simulink model "Test_PQ_Control_LCL_4Legs"  (R2023b)
settings: Solver=VariableStepAuto  StartTime=0.0  StopTime=5  RelTol=1e-3
InitFcn:
  | %Initialization_for_ESS_3P_2L_220kW;
values from neighbouring files (symbols this model uses):
  C_grid = 54e-6    (= 5.4e-05)    [Initialization_for_ESS_3P_2L_220kW.m]    (also in Initialization_for_Testbench.m = 4.5e-05)
  Cdc = 180e-6    (= 0.00018)    [CurrentLoop.m]    (also in Initialization_for_ESS_3P_2L_220kW.m; Initialization_for_Testbench.m)
  Fnom_Grid = 50    [CurrentLoop.m]    (also in Initialization_for_ESS_3P_2L_220kW.m; Initialization_for_Testbench.m)
  L_grid = 200e-6    (= 0.0002)    [Initialization_for_ESS_3P_2L_220kW.m]    (also in Initialization_for_Testbench.m)
  Ts_Control = 62.5e-6    (= 6.25e-05)    [CurrentLoop.m]    (also in Initialization_for_ESS_3P_2L_220kW.m; Initialization_for_Testbench.m = 0.0001)
  Ts_Power = 10e-7    (= 1e-06)    [Initialization_for_ESS_3P_2L_220kW.m]    (also in Initialization_for_Testbench.m)
  Udc_ref = 1500    [CurrentLoop.m]    (also in Initialization_for_ESS_3P_2L_220kW.m; Initialization_for_Testbench.m)
  Unom_Grid = 690    [CurrentLoop.m]    (also in Initialization_for_ESS_3P_2L_220kW.m; Initialization_for_Testbench.m)
undefined symbols (not defined in the file or in its folder): L_neutral
libraries: spsSeriesRLCBranchLib x4, spsThreePhaseVIMeasurementLib x4, simulink x3, spsTriangleGeneratorLib x3, spsThreePhaseSeriesRLCBranchLib x3, spsMultimeterLib x2, spsThreePhaseSeriesRLCLoadLib x2, spsThreePhaseBreakerLib x2, spsUniversalBridgeLib x2, eeStairGenerator x1, spsDCVoltageSourceLib x1, spsRMSLib x1
settings Model: Creator=ZZY  LastModifiedBy=ZZY
settings DataIOCC: ReturnWorkspaceOutputs=off
settings OptimizationCC: UseDivisionForNetSlopeComputation=on

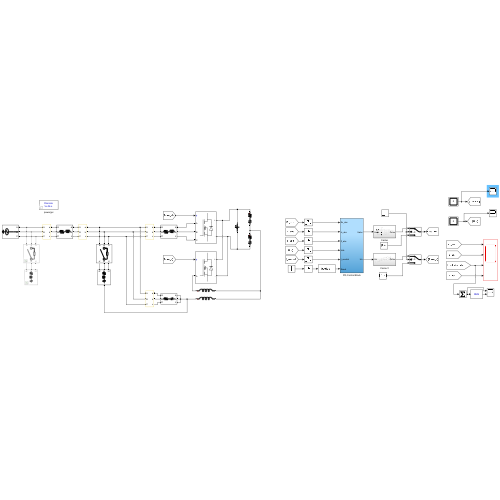
[thumbnail: Simulink's stored preview of the top-level diagram]
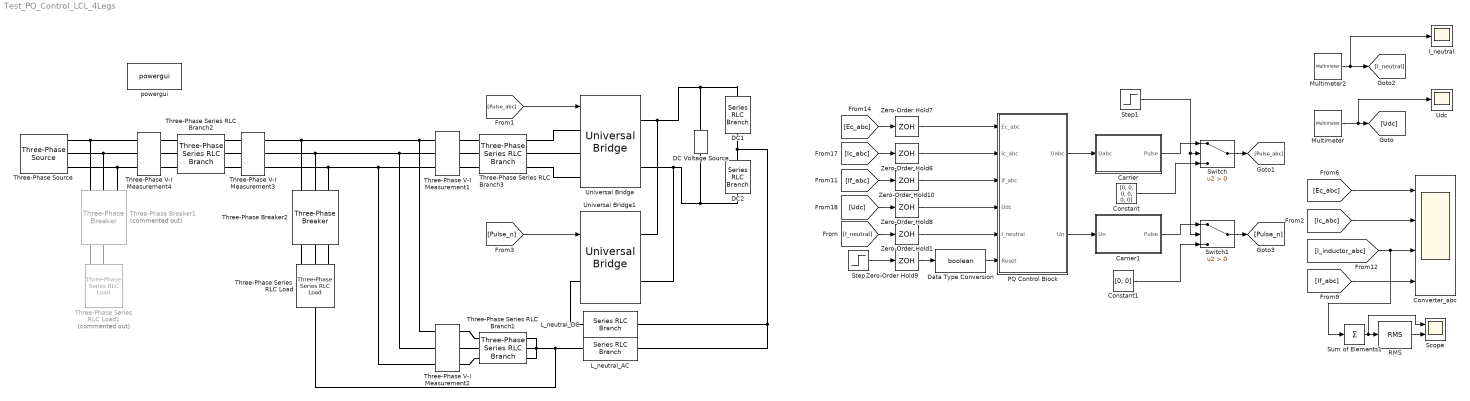
== system Test_PQ_Control_LCL_4Legs ==
  " PQ Control Block" : Subsystem
  Carrier : Subsystem
  Carrier1 : Subsystem
  Constant : Constant  Value=[0, 0, 0, 0, 0, 0]
  Constant1 : Constant  Value=[0, 0]
  Converter_abc : Scope  NumInputPorts=4
  DC Voltage Source : spsDCVoltageSourceLib/DC Voltage Source  Amplitude=Udc_ref  Measurements=None
  DC1 : spsSeriesRLCBranchLib/Series RLC Branch  LConnTagsString=__new0  RConnTagsString=__new0  BranchType=RC  Resistance=1e-4  Inductance=1e-3  SetiL0=off  InitialCurrent=0  Capacitance=Cdc*1.1  Setx0=on  InitialVoltage=Udc_ref/3  Measurements=Branch voltage
  DC2 : spsSeriesRLCBranchLib/Series RLC Branch  LConnTagsString=__new0  RConnTagsString=__new0  BranchType=RC  Resistance=1e-4  Inductance=1e-3  SetiL0=off  InitialCurrent=0  Capacitance=Cdc*0.9  Setx0=on  InitialVoltage=Udc_ref/2  Measurements=Branch voltage
  Data Type Conversion : DataTypeConversion  OutDataTypeStr=boolean  SaturateOnIntegerOverflow=off  RndMeth=Floor
  I_neutral : Scope
  L_neutral_AC : spsSeriesRLCBranchLib/Series RLC Branch  LConnTagsString=__new0  RConnTagsString=__new0  BranchType=L  Resistance=1e-6  Inductance=100e-6  SetiL0=off  InitialCurrent=0  Capacitance=Cdc  Setx0=on  InitialVoltage=750  Measurements=Branch current
  L_neutral_DC : spsSeriesRLCBranchLib/Series RLC Branch  LConnTagsString=__new0  RConnTagsString=__new0  BranchType=L  Resistance=L_neutral  Inductance=L_neutral  SetiL0=off  InitialCurrent=0  Capacitance=Cdc  Setx0=on  InitialVoltage=750  Measurements=Branch current
  Multimeter : spsMultimeterLib/Multimeter  L=4  sel=[1 2]  yselected={}  Gain=[1 1]  OutputType=Complex  PlotAtSimulationStop=off  PhasorSimulation=off
  Multimeter2 : spsMultimeterLib/Multimeter  L=4  sel=[3 4]  yselected={}  Gain=[1 1]  OutputType=Complex  PlotAtSimulationStop=off  PhasorSimulation=off
  RMS : spsRMSLib/RMS  TrueRMS=on  Freq=100  RMSInit=0  Ts=0
  Scope : Scope  NumInputPorts=2
  Step : Step  Time=0.5  OutDataTypeStr=Inherit: Inherit via back propagation  SampleTime=Ts_Control
  Step1 : Step  Time=0.01  OutDataTypeStr=Inherit: Inherit via back propagation  SampleTime=Ts_Control
  Sum of Elements1 : Sum  Inputs=+
  Switch : Switch  Criteria=u2 > Threshold  SaturateOnIntegerOverflow=off  InputSameDT=off
  Switch1 : Switch  Criteria=u2 > Threshold  SaturateOnIntegerOverflow=off  InputSameDT=off
  Three-Phase Series RLC Branch1 : spsThreePhaseSeriesRLCBranchLib/Three-Phase Series RLC Branch  LConnTagsString=A|B|C  RConnTagsString=A|B|C  BranchType=RC  Resistance=10e-3  Inductance=1e-3  Capacitance=C_grid  Measurements=None
  Three-Phase Series RLC Branch2 : spsThreePhaseSeriesRLCBranchLib/Three-Phase Series RLC Branch  LConnTagsString=A|B|C  RConnTagsString=A|B|C  BranchType=RL  Resistance=1e-6  Inductance=L_grid*1  Capacitance=1e-6  Measurements=None
  Three-Phase Series RLC Branch3 : spsThreePhaseSeriesRLCBranchLib/Three-Phase Series RLC Branch  LConnTagsString=A|B|C  RConnTagsString=A|B|C  BranchType=RL  Resistance=1e-6  Inductance=L_grid  Capacitance=1e-6  Measurements=None
  Three-Phase Series RLC Load : spsThreePhaseSeriesRLCLoadLib/Three-Phase Series RLC Load  LConnTagsString=A|B|C  RConnTagsString=N  Configuration=Y (neutral)  NominalVoltage=690  Vabc=[400 400 400]  Vabcp=[1e3 1e3 1e3]  NominalFrequency=50  UnbalancedPower=on  ActivePower=100e3  InductivePower=50e3  CapacitivePower=0  Pabc=[10e3 9e3 11e3]  QLabc=[10 90 110]  QCabc=[100 90 110]  Pabcp=[10e3 9e3 11e3]  QLabcp=[100 90 110]  QCabcp=[100 90 110]  Measurements=None  LoadType=constant Z
  Three-Phase Series RLC Load1 : spsThreePhaseSeriesRLCLoadLib/Three-Phase Series RLC Load  Commented=on  LConnTagsString=A|B|C  Configuration=Delta  NominalVoltage=690  Vabc=[400 400 400]  Vabcp=[1e3 1e3 1e3]  NominalFrequency=50  UnbalancedPower=on  ActivePower=100e3  InductivePower=50e3  CapacitivePower=0  Pabc=[10e3 9e3 11e3]  QLabc=[10 90 110]  QCabc=[100 90 110]  Pabcp=[10e3 9e3 11e3]  QLabcp=[100 90 110]  QCabcp=[100 90 110]  Measurements=None  LoadType=constant Z
  Three-Phase V-I Measurement1 : spsThreePhaseVIMeasurementLib/Three-Phase V-I Measurement  VoltageMeasurement=no  SetLabelV=on  LabelV=Ec_abc  Vpu=off  VpuLL=off  CurrentMeasurement=yes  SetLabelI=on  LabelI=I_inductor_abc  Ipu=off  Pbase=100e6  Vbase=500e3  OutputType=Complex  PhasorSimulation=off  PSBequivalent=0
  Three-Phase V-I Measurement2 : spsThreePhaseVIMeasurementLib/Three-Phase V-I Measurement  VoltageMeasurement=no  SetLabelV=off  LabelV=Ec_abc  Vpu=off  VpuLL=off  CurrentMeasurement=yes  SetLabelI=on  LabelI=If_abc  Ipu=off  Pbase=100e6  Vbase=500e3  OutputType=Complex  PhasorSimulation=off  PSBequivalent=0
  Three-Phase V-I Measurement3 : spsThreePhaseVIMeasurementLib/Three-Phase V-I Measurement  VoltageMeasurement=phase-to-phase  SetLabelV=on  LabelV=Ec_abc  Vpu=off  VpuLL=off  CurrentMeasurement=yes  SetLabelI=on  LabelI=Ic_abc  Ipu=off  Pbase=100e6  Vbase=500e3  OutputType=Complex  PhasorSimulation=off  PSBequivalent=0
  Three-Phase V-I Measurement4 : spsThreePhaseVIMeasurementLib/Three-Phase V-I Measurement  VoltageMeasurement=phase-to-phase  SetLabelV=on  LabelV=Eg_abc  Vpu=off  VpuLL=off  CurrentMeasurement=no  SetLabelI=on  LabelI=Ic_abc  Ipu=off  Pbase=100e6  Vbase=500e3  OutputType=Complex  PhasorSimulation=off  PSBequivalent=0
  Three-Phase Breaker1 : spsThreePhaseBreakerLib/Three-Phase Breaker  Commented=on  InitialState=open  SwitchA=on  SwitchB=on  SwitchC=on  SwitchTimes="[0.9  2.5]"  External=off  BreakerResistance=0.01  SnubberResistance=1e6  SnubberCapacitance=inf  Measurements=None
  Three-Phase Breaker2 : spsThreePhaseBreakerLib/Three-Phase Breaker  InitialState=open  SwitchA=on  SwitchB=on  SwitchC=on  SwitchTimes="[0.9  2.3]"  External=off  BreakerResistance=0.01  SnubberResistance=1e6  SnubberCapacitance=inf  Measurements=None
  Three-Phase Source : spsThreePhaseSourceLib/Three-Phase Source  InternalConnection=Yg  VoltagePhases=off  Voltage=Unom_Grid  PhaseAngle=0  Voltage_phases=[25e3 25e3 25e3]/sqrt(3)  PhaseAngles_phases=[0 -120 +120]  Frequency=Fnom_Grid  NonIdealSource=off  SpecifyImpedance=off  Resistance=1e-3  Inductance=400e-6  ShortCircuitLevel=100e6  BaseVoltage=Unom_Grid  XRratio=7  BusType=swing  Pref=10e3  Qref=0  Prefabc=[10e3, 10e3, 10e3]  Qrefabc=[0, 0, 0]  Qmin=-inf  Qmax=inf
  Udc : Scope
  Universal Bridge : spsUniversalBridgeLib/Universal Bridge  Arms=3  SnubberResistance=1e5  SnubberCapacitance=inf  Device=MOSFET / Diodes  Ron=1e-3  Lon=0  ForwardVoltages="[  0  0  ]"  ForwardVoltage=0  GTOparameters=[ 10e-6 , 20e-6 ]  IGBTparameters=[ 1e-6 , 2e-6 ]  Measurements=None  Measurements_2=None  converterType=Rectifier
  Universal Bridge1 : spsUniversalBridgeLib/Universal Bridge  Arms=1  SnubberResistance=1e5  SnubberCapacitance=inf  Device=MOSFET / Diodes  Ron=1e-3  Lon=0  ForwardVoltages="[  0  0  ]"  ForwardVoltage=0  GTOparameters=[ 10e-6 , 20e-6 ]  IGBTparameters=[ 1e-6 , 2e-6 ]  Measurements=None  Measurements_2=None  converterType=Rectifier
  Zero-Order Hold{1,6..10} (6 alike) : ZeroOrderHold  SampleTime=Ts_Control
  powergui : spspowerguiLib/powergui  Priority=1  SimulationMode=Discrete  SampleTime=Ts_Power  frequency=60  Iterations=50  frequencyindice=50  Pbase=100e6  ErrMax=1e-4  UnitsV=kV  UnitsW=MW  buscounter=0  FunctionMessages=off  echomessages=off  EnableUseOfTLC=off  CurrentSourceSwitches=off  DisableSnubberDevices=off  DisableRonSwitches=off  DisableVfSwitches=off  DisplayEquations=off  AutomaticDiscreteSolvers=off  SolverType=Tustin/Backward Euler (TBE)  Interpol=off  ExternalGateDelay=off  methode=off  Ts=100  x0status=blocks  SPID=on  SwTol=0  HookPort=off  NonlinearTolerance=1e-4  nMaxIteration=100  ContinueOnMaxIteration=off  RestoreLinks=warning  ResistiveCurrentMeasurement=off  Frange=[0:2:500]  Ylog=off  Xlog=on  ShowGrid=off  save=off  variable=ZData  structure=CHB_abc  ZoomFFT=off  StartTime=1.4  cycles=5  DisplayStyle=1  fundamental=50  FreqAxis=off  MaxFrequency=30000  frequencyindicesteady=1  RmsSteady=1  display=off
  wires:
  [Ec_abc] -> Converter_abc/1
  [Ic_abc] -> Converter_abc/2
  [Pulse_abc] -> Universal Bridge/1
  [Ec_abc] -> Zero-Order Hold7/1
  [Ic_abc] -> Zero-Order Hold6/1
  [Udc] -> Zero-Order Hold8/1
  Zero-Order Hold8/1 -> " PQ Control Block"/4(Udc)
  Step/1 -> Zero-Order Hold9/1
  Carrier/1(Pulse) -> Switch/1
  Data Type Conversion/1 -> " PQ Control Block"/6(Reset)
  Zero-Order Hold9/1 -> Data Type Conversion/1
  Zero-Order Hold6/1 -> " PQ Control Block"/2(Ic_abc)
  Zero-Order Hold7/1 -> " PQ Control Block"/1(Ec_abc)
  [If_abc] -> Converter_abc/4
  [If_abc] -> Zero-Order Hold10/1
  Zero-Order Hold10/1 -> " PQ Control Block"/3(If_abc)
  RMS/1 -> Scope/2
  [I_inductor_abc] -> Sum of Elements1/1, Converter_abc/3
  " PQ Control Block"/1(Uabc) -> Carrier/1(Uabc)
  Sum of Elements1/1 -> Scope/1, RMS/1
  Multimeter/1 -> Udc/1, [Udc]
  Zero-Order Hold1/1 -> " PQ Control Block"/5(I_neutral)
  [I_neutral] -> Zero-Order Hold1/1
  " PQ Control Block"/2(Un) -> Carrier1/1(Un)
  Carrier1/1(Pulse) -> Switch1/1
  [Pulse_n] -> Universal Bridge1/1
  Multimeter2/1 -> [I_neutral], I_neutral/1
  Switch/1 -> [Pulse_abc]
  Switch1/1 -> [Pulse_n]
  Step1/1 -> Switch1/2, Switch/2
  Constant/1 -> Switch/3
  Constant1/1 -> Switch1/3
  connections:
  Three-Phase V-I Measurement1/LConn1 -- Three-Phase V-I Measurement2/LConn1 -- Three-Phase Breaker2/RConn1 -- Three-Phase V-I Measurement3/RConn1
  Three-Phase V-I Measurement1/LConn2 -- Three-Phase V-I Measurement2/LConn2 -- Three-Phase Breaker2/RConn2 -- Three-Phase V-I Measurement3/RConn2
  Three-Phase V-I Measurement1/LConn3 -- Three-Phase V-I Measurement2/LConn3 -- Three-Phase Breaker2/RConn3 -- Three-Phase V-I Measurement3/RConn3
  DC1/LConn1 -- Universal Bridge/RConn1 -- Universal Bridge1/RConn1 -- DC Voltage Source/RConn1
  Three-Phase V-I Measurement1/RConn1 -- Three-Phase Series RLC Branch3/LConn1
  Three-Phase V-I Measurement1/RConn2 -- Three-Phase Series RLC Branch3/LConn2
  Three-Phase V-I Measurement1/RConn3 -- Three-Phase Series RLC Branch3/LConn3
  Three-Phase Source/RConn3 -- Three-Phase Breaker1/RConn3 -- Three-Phase V-I Measurement4/LConn3
  Three-Phase Source/RConn2 -- Three-Phase Breaker1/RConn2 -- Three-Phase V-I Measurement4/LConn2
  Three-Phase Source/RConn1 -- Three-Phase Breaker1/RConn1 -- Three-Phase V-I Measurement4/LConn1
  Three-Phase Breaker2/LConn1 -- Three-Phase Series RLC Load/LConn1
  Three-Phase Breaker2/LConn2 -- Three-Phase Series RLC Load/LConn2
  Three-Phase Breaker2/LConn3 -- Three-Phase Series RLC Load/LConn3
  Three-Phase Series RLC Branch1/LConn2 -- Three-Phase V-I Measurement2/RConn2
  Three-Phase V-I Measurement2/RConn1 -- Three-Phase Series RLC Branch1/LConn1
  Three-Phase V-I Measurement2/RConn3 -- Three-Phase Series RLC Branch1/LConn3
  Three-Phase Series RLC Branch1/RConn1 -- L_neutral_AC/LConn1 -- Three-Phase Series RLC Load/RConn1 -- Three-Phase Series RLC Branch1/RConn3 -- Three-Phase Series RLC Branch1/RConn2
  Three-Phase Series RLC Branch2/RConn1 -- Three-Phase V-I Measurement3/LConn1
  Three-Phase Series RLC Branch2/RConn2 -- Three-Phase V-I Measurement3/LConn2
  Three-Phase Series RLC Branch2/RConn3 -- Three-Phase V-I Measurement3/LConn3
  Three-Phase V-I Measurement4/RConn1 -- Three-Phase Series RLC Branch2/LConn1
  Three-Phase V-I Measurement4/RConn2 -- Three-Phase Series RLC Branch2/LConn2
  Three-Phase V-I Measurement4/RConn3 -- Three-Phase Series RLC Branch2/LConn3
  Three-Phase Series RLC Branch3/RConn2 -- Universal Bridge/LConn2
  Universal Bridge/LConn1 -- Three-Phase Series RLC Branch3/RConn1
  Three-Phase Series RLC Branch3/RConn3 -- Universal Bridge/LConn3
  DC2/RConn1 -- Universal Bridge/RConn2 -- Universal Bridge1/RConn2 -- DC Voltage Source/LConn1
  DC1/RConn1 -- L_neutral_AC/RConn1 -- L_neutral_DC/RConn1 -- DC2/LConn1
  L_neutral_DC/LConn1 -- Universal Bridge1/LConn1
  Three-Phase Breaker1/LConn1 -- Three-Phase Series RLC Load1/LConn1
  Three-Phase Breaker1/LConn2 -- Three-Phase Series RLC Load1/LConn2

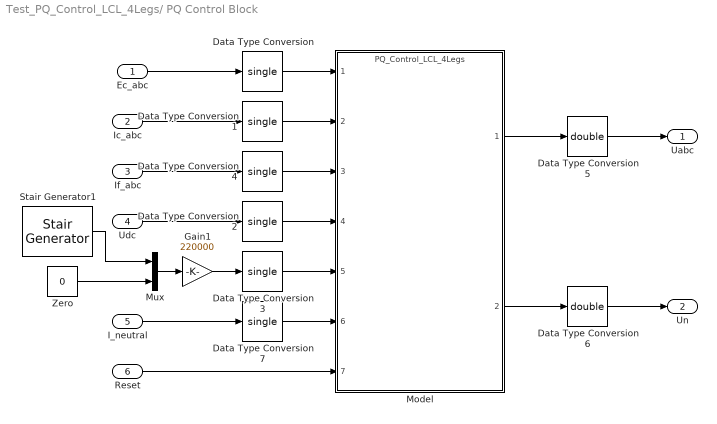
== system Test_PQ_Control_LCL_4Legs/ PQ Control Block ==
  Ec_abc : Inport
  Ic_abc : Inport  Port=2
  If_abc : Inport  Port=3
  Udc : Inport  Port=4
  I_neutral : Inport  Port=5
  Reset : Inport  Port=6  OutDataTypeStr=boolean
  Data Type Conversion{,1..4,7} (6 alike) : DataTypeConversion  OutDataTypeStr=single  RndMeth=Nearest  SaturateOnIntegerOverflow=off
  Data Type Conversion5 : DataTypeConversion  OutDataTypeStr=double  RndMeth=Nearest  SaturateOnIntegerOverflow=off
  Data Type Conversion6 : DataTypeConversion  OutDataTypeStr=double  RndMeth=Nearest  SaturateOnIntegerOverflow=off
  Gain1 : Gain  Gain=220000
  Model : ModelReference  ModelNameDialog=PQ_Control_LCL_4Legs.slx  SimulationMode=Normal  ModelReferenceVersion=1.105
  Mux : Mux  Inputs=2
  Stair Generator1 : eeStairGenerator/Stair Generator  LabelModeActiveChoice=Discrete  TimeInput=0:0.5:5  AmplitudeInput=0:0.1:1  SampleTime=Ts_Control  RepeatPattern=off  OutDataTypeStr=double
      settings: LibrarySourceBlock=ee_sl_lib/General Control/Stair Generator
  Zero : Constant  Value=0  OutDataTypeStr=Inherit: Inherit via back propagation
  Uabc : Outport
  Un : Outport  Port=2
  wires:
  Ec_abc/1 -> Data Type Conversion/1
  Ic_abc/1 -> Data Type Conversion1/1
  Udc/1 -> Data Type Conversion2/1
  Model/1 -> Data Type Conversion5/1
  Stair Generator1/1 -> Mux/1
  Zero/1 -> Mux/2
  Data Type Conversion/1 -> Model/1
  Data Type Conversion1/1 -> Model/2
  Data Type Conversion5/1 -> Uabc/1
  Reset/1 -> Model/7
  Mux/1 -> Gain1/1
  Data Type Conversion3/1 -> Model/5
  Data Type Conversion2/1 -> Model/4
  Gain1/1 -> Data Type Conversion3/1
  If_abc/1 -> Data Type Conversion4/1
  Data Type Conversion4/1 -> Model/3
  Data Type Conversion6/1 -> Un/1
  Model/2 -> Data Type Conversion6/1
  I_neutral/1 -> Data Type Conversion7/1
  Data Type Conversion7/1 -> Model/6

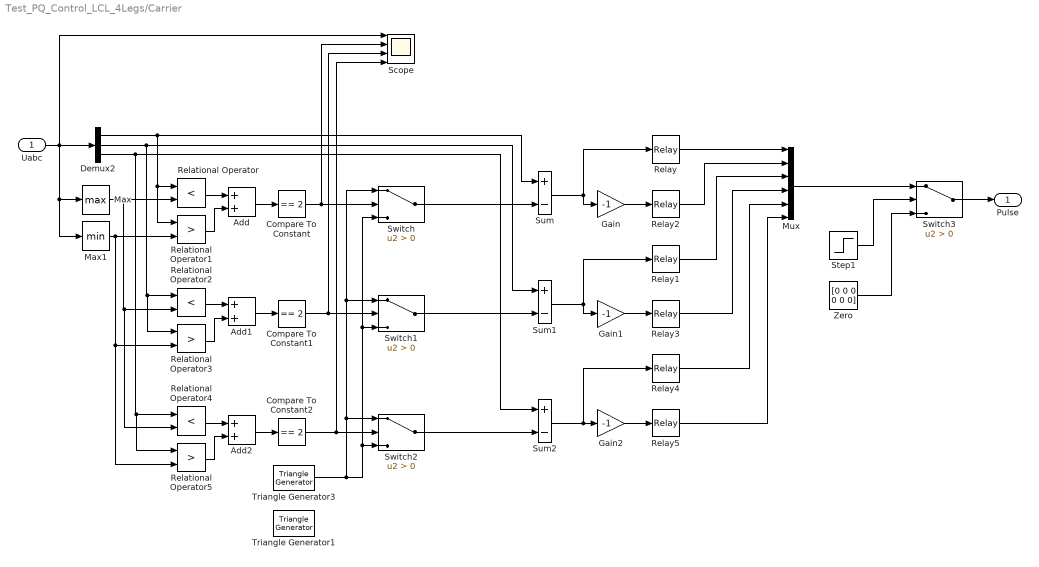
== system Test_PQ_Control_LCL_4Legs/Carrier ==
  Uabc : Inport
  Add : Sum
  Add1 : Sum
  Add2 : Sum
  Compare To Constant : simulink/Logic and Bit Operations/Compare To Constant  relop===  const=2  OutDataTypeStr=boolean
  Compare To Constant1 : simulink/Logic and Bit Operations/Compare To Constant  relop===  const=2  OutDataTypeStr=boolean
  Compare To Constant2 : simulink/Logic and Bit Operations/Compare To Constant  relop===  const=2  OutDataTypeStr=boolean
  Demux2 : Demux  Outputs=3
  Gain : Gain  Gain=-1
  Gain1 : Gain  Gain=-1
  Gain2 : Gain  Gain=-1
  Max : MinMax  Function=max
  Max1 : MinMax
  Mux : Mux  Inputs=6
  Relational Operator : RelationalOperator  Operator=<  OutDataTypeStr=boolean  RndMeth=Simplest  InputSameDT=off
  Relational Operator1 : RelationalOperator  Operator=>  OutDataTypeStr=boolean  RndMeth=Simplest  InputSameDT=off
  Relational Operator2 : RelationalOperator  Operator=<  OutDataTypeStr=boolean  RndMeth=Simplest  InputSameDT=off
  Relational Operator3 : RelationalOperator  Operator=>  OutDataTypeStr=boolean  RndMeth=Simplest  InputSameDT=off
  Relational Operator4 : RelationalOperator  Operator=<  OutDataTypeStr=boolean  RndMeth=Simplest  InputSameDT=off
  Relational Operator5 : RelationalOperator  Operator=>  OutDataTypeStr=boolean  RndMeth=Simplest  InputSameDT=off
  Relay{,1..5} (6 alike) : Relay  OffSwitchValue=-eps
  Scope : Scope  NumInputPorts=4
  Step1 : Step  Time=0.001  OutDataTypeStr=Inherit: Inherit via back propagation
  Sum : Sum  Inputs=+-
  Sum1 : Sum  Inputs=+-
  Sum2 : Sum  Inputs=+-
  Switch{,1..3} (4 alike) : Switch  Criteria=u2 > Threshold  SaturateOnIntegerOverflow=off  InputSameDT=off
  Triangle Generator1 : spsTriangleGeneratorLib/Triangle Generator  Freq=16000  Phase=0  Ts=1e-6
  Triangle Generator3 : spsTriangleGeneratorLib/Triangle Generator  Freq=16000  Phase=180  Ts=1e-6
  Zero : Constant  Value=[0 0 0 0 0 0]  OutDataTypeStr=Inherit: Inherit via back propagation
  Pulse : Outport
  wires:
  Gain/1 -> Relay2/1
  Sum/1 -> Relay/1, Gain/1
  Switch/1 -> Sum/2
  Uabc/1 -> Scope/1, Max1/1, Max/1, Demux2/1
  Demux2/1 -> Sum/1, Relational Operator1/1, Relational Operator/1
  Relay/1 -> Mux/1
  Relay2/1 -> Mux/2
  Relay1/1 -> Mux/3
  Relay3/1 -> Mux/4
  Gain1/1 -> Relay3/1
  Demux2/2 -> Relational Operator3/1, Relational Operator2/1, Sum1/1
  Sum1/1 -> Relay1/1, Gain1/1
  Switch1/1 -> Sum1/2
  Relay5/1 -> Mux/6
  Demux2/3 -> Relational Operator5/1, Relational Operator4/1, Sum2/1
  Gain2/1 -> Relay5/1
  Sum2/1 -> Relay4/1, Gain2/1
  Switch2/1 -> Sum2/2
  Relay4/1 -> Mux/5
  Triangle Generator3/1 -> Switch2/3, Switch1/3, Switch/3, Switch/1, Switch1/1, Switch2/1
  Compare To Constant/1 -> Scope/2, Switch/2
  Compare To Constant1/1 -> Scope/3, Switch1/2
  Compare To Constant2/1 -> Scope/4, Switch2/2
  Add/1 -> Compare To Constant/1
  Add1/1 -> Compare To Constant1/1
  Add2/1 -> Compare To Constant2/1
  Relational Operator/1 -> Add/1
  Relational Operator1/1 -> Add/2
  Max/1 -> Relational Operator4/2, Relational Operator2/2, Relational Operator/2
  Max1/1 -> Relational Operator5/2, Relational Operator3/2, Relational Operator1/2
  Relational Operator2/1 -> Add1/1
  Relational Operator3/1 -> Add1/2
  Relational Operator4/1 -> Add2/1
  Relational Operator5/1 -> Add2/2
  Step1/1 -> Switch3/2
  Mux/1 -> Switch3/1
  Zero/1 -> Switch3/3
  Switch3/1 -> Pulse/1

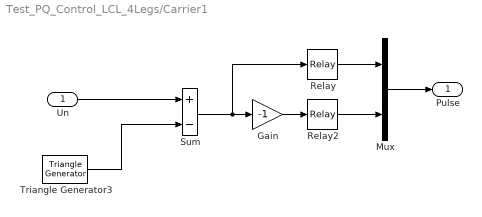
== system Test_PQ_Control_LCL_4Legs/Carrier1 ==
  Un : Inport
  Gain : Gain  Gain=-1
  Mux : Mux  Inputs=2
  Relay : Relay  OffSwitchValue=-eps
  Relay2 : Relay  OffSwitchValue=-eps
  Sum : Sum  Inputs=+-
  Triangle Generator3 : spsTriangleGeneratorLib/Triangle Generator  Freq=16000  Phase=180  Ts=1e-6
  Pulse : Outport
  wires:
  Gain/1 -> Relay2/1
  Sum/1 -> Relay/1, Gain/1
  Triangle Generator3/1 -> Sum/2
  Relay/1 -> Mux/1
  Relay2/1 -> Mux/2
  Mux/1 -> Pulse/1
  Un/1 -> Sum/1
